simulink model "sim_comparison"  (R2016b)
settings: Solver=ode3  StartTime=0.0  StopTime=Tsim  FixedStep=Ts  RelTol=1e-3  EnableMultiTasking=on
values from neighbouring files (symbols this model uses):
  C_meas = [zeros(ny,3) eye(ny)]    [run_sim.m]
  C_scope = [eye(2) zeros(2,1+ny)]    [run_sim.m]
  dist = 2e-2    (= 0.02)    [run_sim.m]
  P = ss(A,[Bw Bu],[Cz;Cy],[Dzw Dzu; Dyw zeros(size(Cy,1),1)])    [system_def.m]
  ref = 1    [run_sim.m]
  Tdist = 15    [run_sim.m]
  Tref = 2    [run_sim.m]
  x0 = [0;zeros(size(P.A,1)-1,1)]    [run_sim.m]
undefined symbols (not defined in the file or in its folder): Kcomp, xKcomp0
settings Model: Creator=Matti  LastModifiedBy=user
settings OptimizationCC: LifeSpan=inf
settings DebuggingCC: SFUnexpectedBacktrackingDiag=warning  SFNoUnconditionalDefaultTransitionDiag=warning  SFExecutionAtInitializationDiag=none
settings GRTTargetCC: TargetLangStandard=C89/C90 (ANSI)  GeneratePreprocessorConditionals=Disable all
settings ConfigComp: CovMetricSettings=dw  CovHtmlReporting=on  CovSaveCumulativeToWorkspaceVar=on  CovSaveSingleToWorkspaceVar=on  CovExternalEMLEnable=off

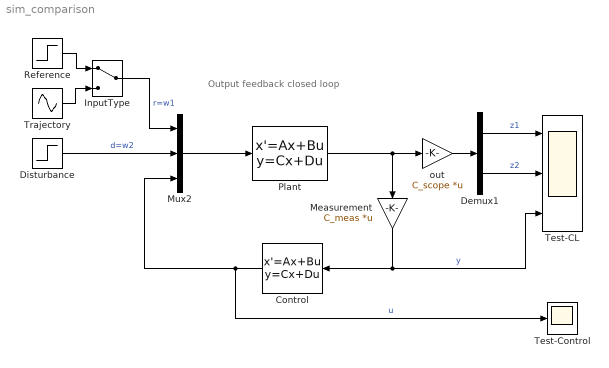
== system sim_comparison ==
  note: Output feedback closed loop
  Control : StateSpace  A=Kcomp.A  B=Kcomp.B  C=Kcomp.C  D=Kcomp.D  X0=xKcomp0
  Demux1 : Demux  Outputs=2
  Disturbance : Step  Time=Tdist  After=dist  SampleTime=0
  InputType : ManualSwitch
  Measurement : Gain  Gain=C_meas  Multiplication=Matrix(K*u)
  Mux2 : Mux  Inputs=3
  Plant : StateSpace  A=P.A  B=P.B  C=P.C  D=P.D  X0=x0
  Reference : Step  Time=Tref  After=ref  SampleTime=0
  Test-CL : Scope  NumInputPorts=3
  Test-Control : Scope
  Trajectory : Sin  Frequency=0.5  SampleTime=0
  out : Gain  Gain=C_scope  Multiplication=Matrix(K*u)
  wires:
  Disturbance/1 -> Mux2/2  "d=w2"
  Measurement/1 -> Test-CL/3, Control/1  "y"
  Plant/1 -> Measurement/1, out/1
  Control/1 -> Test-Control/1, Mux2/3  "u"
  Mux2/1 -> Plant/1
  Reference/1 -> InputType/1
  InputType/1 -> Mux2/1  "r=w1"
  Trajectory/1 -> InputType/2
  Demux1/1 -> Test-CL/1  "z1"
  out/1 -> Demux1/1
  Demux1/2 -> Test-CL/2  "z2"
